simulink model "Ver1"  (R2025a)
settings: Solver=VariableStepAuto  StartTime=0.0  StopTime=50  RelTol=1e-3
model workspace (MAT data in the model file):
  params : Simulink.Parameter (value not decoded)
values from neighbouring files (symbols this model uses):
  edges = getappdata(0, 'DataEdges')    [DataAnalysis.m]    (also in Data_Analysis.m = graph_params.edges; Trajectory.m = getappdata(0, 'Edges'); data.m = graph_params.edges; formation_data.mat = [1 1 1 1 1 1 1 1 1 1 2 3 ... (62 elements, 31x2)])
  p10_init = [9; 5; 0]    [data.m]
  p2_init = [10; 0; 0]    [data.m]
  p3_init = [0; 10; 0]    [data.m]
  p4_init = [-10; 0; 0]    [data.m]
  p5_init = [0; -10; 0]    [data.m]
  p6_init = [7; 7; 0]    [data.m]
  p7_init = [-7; 7; 0]    [data.m]
  p8_init = [-7; -7; 0]    [data.m]
  p9_init = [7; -7; 0]    [data.m]
(part 2 of 3)

== matlab function Ver1/Drone 6/MATLAB Function1 ==
  data: p input; pes input; v input; u output; params parameter Bus: params_bus
function u = fcn(p, pes, v, params)

    graph_params = params.graph_params;
    formation_params = params.formation_params;
    conn_params = params.conn_params;
    avoid_params = params.avoid_params;
    prior_params = params.prior_params;

    % Chuyển vector p thành mảng 3x5
    pos = reshape(p, 3, graph_params.n_drones);
    vel = reshape(v, 3, graph_params.n_drones);
    pes = reshape(pes, 3, graph_params.n_drones);
    
    n_edges = size(graph_params.edges, 1);
    

    i_drone = 6;
    
    % =====================================================================
    %  FORMATION CONTROL (Distance-based + Backstepping)
    % =====================================================================
    u_form = zeros(3,1);
    gradV = zeros(3,1);
    dgradV = zeros(3,1);
    
    for e = 1:n_edges
        if graph_params.edges(e,1) == i_drone
            j = graph_params.edges(e,2);
            p_ij = pos(:,j) - pos(:,i_drone);
            v_ij = vel(:,j) - vel(:,i_drone);
            dij = norm(p_ij);
            
            if dij > 1e-6
                e_ij = dij^2 - formation_params.d_star(e)^2;
                
                % Lực formation (gradient descent)
                u_form = u_form + formation_params.alpha * e_ij * p_ij;
                
                % Gradient V
                gradV = gradV + e_ij * p_ij;
                
                % Đạo hàm gradient V
                term = 2*(p_ij' * v_ij) * p_ij + e_ij * v_ij;
                dgradV = dgradV + term;
            end
            
        elseif graph_params.edges(e,2) == i_drone
            j = graph_params.edges(e,1);
            p_ij = pos(:,j) - pos(:,i_drone);
            v_ij = vel(:,j) - vel(:,i_drone);
            dij = norm(p_ij);
            
            if dij > 1e-6
                e_ij = dij^2 - formation_params.d_star(e)^2;
                
                u_form = u_form + formation_params.alpha * e_ij * p_ij;
                gradV = gradV + e_ij * p_ij;
                term = 2*(p_ij' * v_ij) * p_ij + e_ij * v_ij;
                dgradV = dgradV + term;
            end
        end
    end
    
    % Giới hạn gradient
    gradV = max(min(gradV, 15), -15);
    dgradV = max(min(dgradV, 20), -20);
    
    % Backstepping
    u_back = -formation_params.kp * gradV - formation_params.kd * dgradV;
    
    % Damping
    v_i = vel(:,i_drone);
    u_damp = -formation_params.beta * v_i;
    
    % =====================================================================
    %  CONNECTIVITY MAINTENANCE
    % =====================================================================
    % Tính ma trận kề sigmoid
    A = zeros(graph_params.n_drones);
    for i = 1:graph_params.n_drones
        for j = i+1:graph_params.n_drones
            d_ij = norm(pos(:,i) - pos(:,j));
            a_ij = 1 / (1 + exp(-conn_params.omega * (conn_params.d_max - d_ij)));
            A(i,j) = a_ij;
            A(j,i) = a_ij;
        end
    end
    
    % Ma trận Laplace
    D = diag(sum(A,2));
    L = D - A;
    
    % Tính M = Q'*L*Q
    Q = conn_params.Q;
    M = Q' * L * Q;
    lambda2 = min(eig(M));
    
    detM = det(M);
    if detM < 1e-6
        detM = 1e-6;
    end
    
    % Tính lực giữ liên kết bằng sai phân số
    u_conn = zeros(3, 1);
    eps_fd = 1e-4;
    
    for d = 1:graph_params.dim
        % M tại p + eps
        pos_plus = pos;
        pos_plus(d, i_drone) = pos_plus(d, i_drone) + eps_fd;
        
        A_plus = zeros(graph_params.n_drones);
        for i = 1:graph_params.n_drones
            for j = i+1:graph_params.n_drones
                d_ij = norm(pos_plus(:,i) - pos_plus(:,j));
                a_ij = 1 / (1 + exp(-conn_params.omega * (conn_params.d_max - d_ij)));
                A_plus(i,j) = a_ij;
                A_plus(j,i) = a_ij;
            end
        end
        D_plus = diag(sum(A_plus,2));
        L_plus = D_plus - A_plus;
        M_plus = Q' * L_plus * Q;
        
        % M tại p - eps
        pos_minus = pos;
        pos_minus(d, i_drone) = pos_minus(d, i_drone) - eps_fd;
        
        A_minus = zeros(graph_params.n_drones);
        for i = 1:graph_params.n_drones
            for j = i+1:graph_params.n_drones
                d_ij = norm(pos_minus(:,i) - pos_minus(:,j));
                a_ij = 1 / (1 + exp(-conn_params.omega * (conn_params.d_max - d_ij)));
                A_minus(i,j) = a_ij;
                A_minus(j,i) = a_ij;
            end
        end
        D_minus = diag(sum(A_minus,2));
        L_minus = D_minus - A_minus;
        M_minus = Q' * L_minus * Q;
        
        dM_dp = (M_plus - M_minus) / (2*eps_fd);
        
        if rcond(M) > 1e-6
            u_conn(d) = conn_params.alpha * trace(M \ dM_dp) / detM^conn_params.alpha;
        else
            u_conn(d) = 0;
        end
    end
    
    % =====================================================================
    %  OBSTACLE AVOIDANCE
    % =====================================================================
    muy = (1 + avoid_params.d_safe^4) / avoid_params.d_safe^4;
    
    % Tính beta_product
    beta_product = 1;
    for e = 1:n_edges
        i = graph_params.edges(e,1);
        j = graph_params.edges(e,2);
        dij = norm(pos(:,i) - pos(:,j));
        beta_val = beta_slide(dij, avoid_params.d_safe, muy);
        beta_product = beta_product * beta_val;
    end
    
    Phi = 1 / (beta_product^avoid_params.alpha);
    dPhi_dbeta = -avoid_params.alpha * beta_product^(-avoid_params.alpha-1);
    
    % Tính lực tránh
    u_avoid = zeros(3, 1);
    eps_deriv = 1e-4;
    
    for j = 1:graph_params.n_drones
        if j == i_drone
            continue;
        end
        
        p_ij = pos(:,i_drone) - pos(:,j);
        dij_ij = norm(p_ij);
        
        if dij_ij > 1e-6
            dd_dp = p_ij;
            
            % Đạo hàm số của beta
            beta_plus = beta_slide(dij_ij + eps_deriv, avoid_params.d_safe, muy);
            beta_minus = beta_slide(dij_ij - eps_deriv, avoid_params.d_safe, muy);
            dbeta_dd = (beta_plus - beta_minus) / (2*eps_deriv);
            
            grad = dPhi_dbeta * dbeta_dd * dd_dp;
            u_avoid = u_avoid - avoid_params.k * grad;
        end
    end
    
    u_h = [0; 0; -prior_params.k_height * (pes(3, i_drone) - pos(3, 1))];


    % =====================================================================
    %  TỔNG HỢP
    % =====================================================================
    u = 5*u_form + u_back + u_damp + 0.5*u_conn + 10*u_avoid + u_h;

end

function beta = beta_slide(dist, d_safe, muy)
    if (dist^2 - d_safe^2) >= 0
        rho = 0;
    else
        rho = 1;
    end
    diff_sq = (dist^2 - d_safe^2)^2;
    beta = (1 - muy * diff_sq / (1 + diff_sq))^rho;
    % Đảm bảo beta không âm
    beta = max(beta, 0);
end

== matlab function Ver1/Drone 6/Pos Estimation ==
  data: p input; v input; pes input; pes_dot output size=[3,1]; params parameter Bus: params_bus
function pes_dot = fcn(p, v, pes, params)

    graph_params = params.graph_params;
    estimation_params = params.estimation_params;

    pes_dot = zeros(3,1);
    
    
    i_drone = 6;  % Drone đang xét
    
    % Reshape input
    pos = reshape(p, graph_params.dim, graph_params.n_drones);
    pes = reshape(pes, graph_params.dim, graph_params.n_drones);
    vel = reshape(v, graph_params.dim, graph_params.n_drones);
    
    % Tính toán gradient term
    grad_term = zeros(graph_params.dim, 1);
    
    n_edges = size(graph_params.edges, 1);
    
    for e = 1:n_edges
        if graph_params.edges(e,1) == i_drone
            j = graph_params.edges(e,2);
        else
            j = graph_params.edges(e,1);
        end

        if j == 1
            grad_term = grad_term + ((pos(:, j) - pes(:,i_drone)) - (pos(:, j) - pos(:, i_drone)));
        else
            grad_term = grad_term + (pes(:, j) - pes(:, i_drone) - (pos(:, j) - pos(:, i_drone)));
        end
    end

    
    % Output
    
    pes_dot1 = vel(:, i_drone) + estimation_params.mu*grad_term;
    pes_dot = [pes_dot1(1); pes_dot1(2); pes_dot1(3)];
end

== matlab function Ver1/Drone 6/Subsystem/Kinematic ==
  data: p_ddot output; u input
function p_ddot = fcn(u)

    p_ddot = u;

end

== matlab function Ver1/Drone 7/MATLAB Function1 ==
  data: p input; pes input; v input; u output; params parameter Bus: params_bus
function u = fcn(p, pes, v, params)

    graph_params = params.graph_params;
    formation_params = params.formation_params;
    conn_params = params.conn_params;
    avoid_params = params.avoid_params;
    prior_params = params.prior_params;

    % Chuyển vector p thành mảng 3x5
    pos = reshape(p, 3, graph_params.n_drones);
    vel = reshape(v, 3, graph_params.n_drones);
    pes = reshape(pes, 3, graph_params.n_drones);
    
    n_edges = size(graph_params.edges, 1);
    

    i_drone = 7;
    
    % =====================================================================
    %  FORMATION CONTROL (Distance-based + Backstepping)
    % =====================================================================
    u_form = zeros(3,1);
    gradV = zeros(3,1);
    dgradV = zeros(3,1);
    
    for e = 1:n_edges
        if graph_params.edges(e,1) == i_drone
            j = graph_params.edges(e,2);
            p_ij = pos(:,j) - pos(:,i_drone);
            v_ij = vel(:,j) - vel(:,i_drone);
            dij = norm(p_ij);
            
            if dij > 1e-6
                e_ij = dij^2 - formation_params.d_star(e)^2;
                
                % Lực formation (gradient descent)
                u_form = u_form + formation_params.alpha * e_ij * p_ij;
                
                % Gradient V
                gradV = gradV + e_ij * p_ij;
                
                % Đạo hàm gradient V
                term = 2*(p_ij' * v_ij) * p_ij + e_ij * v_ij;
                dgradV = dgradV + term;
            end
            
        elseif graph_params.edges(e,2) == i_drone
            j = graph_params.edges(e,1);
            p_ij = pos(:,j) - pos(:,i_drone);
            v_ij = vel(:,j) - vel(:,i_drone);
            dij = norm(p_ij);
            
            if dij > 1e-6
                e_ij = dij^2 - formation_params.d_star(e)^2;
                
                u_form = u_form + formation_params.alpha * e_ij * p_ij;
                gradV = gradV + e_ij * p_ij;
                term = 2*(p_ij' * v_ij) * p_ij + e_ij * v_ij;
                dgradV = dgradV + term;
            end
        end
    end
    
    % Giới hạn gradient
    gradV = max(min(gradV, 15), -15);
    dgradV = max(min(dgradV, 20), -20);
    
    % Backstepping
    u_back = -formation_params.kp * gradV - formation_params.kd * dgradV;
    
    % Damping
    v_i = vel(:,i_drone);
    u_damp = -formation_params.beta * v_i;
    
    % =====================================================================
    %  CONNECTIVITY MAINTENANCE
    % =====================================================================
    % Tính ma trận kề sigmoid
    A = zeros(graph_params.n_drones);
    for i = 1:graph_params.n_drones
        for j = i+1:graph_params.n_drones
            d_ij = norm(pos(:,i) - pos(:,j));
            a_ij = 1 / (1 + exp(-conn_params.omega * (conn_params.d_max - d_ij)));
            A(i,j) = a_ij;
            A(j,i) = a_ij;
        end
    end
    
    % Ma trận Laplace
    D = diag(sum(A,2));
    L = D - A;
    
    % Tính M = Q'*L*Q
    Q = conn_params.Q;
    M = Q' * L * Q;
    lambda2 = min(eig(M));
    
    detM = det(M);
    if detM < 1e-6
        detM = 1e-6;
    end
    
    % Tính lực giữ liên kết bằng sai phân số
    u_conn = zeros(3, 1);
    eps_fd = 1e-4;
    
    for d = 1:graph_params.dim
        % M tại p + eps
        pos_plus = pos;
        pos_plus(d, i_drone) = pos_plus(d, i_drone) + eps_fd;
        
        A_plus = zeros(graph_params.n_drones);
        for i = 1:graph_params.n_drones
            for j = i+1:graph_params.n_drones
                d_ij = norm(pos_plus(:,i) - pos_plus(:,j));
                a_ij = 1 / (1 + exp(-conn_params.omega * (conn_params.d_max - d_ij)));
                A_plus(i,j) = a_ij;
                A_plus(j,i) = a_ij;
            end
        end
        D_plus = diag(sum(A_plus,2));
        L_plus = D_plus - A_plus;
        M_plus = Q' * L_plus * Q;
        
        % M tại p - eps
        pos_minus = pos;
        pos_minus(d, i_drone) = pos_minus(d, i_drone) - eps_fd;
        
        A_minus = zeros(graph_params.n_drones);
        for i = 1:graph_params.n_drones
            for j = i+1:graph_params.n_drones
                d_ij = norm(pos_minus(:,i) - pos_minus(:,j));
                a_ij = 1 / (1 + exp(-conn_params.omega * (conn_params.d_max - d_ij)));
                A_minus(i,j) = a_ij;
                A_minus(j,i) = a_ij;
            end
        end
        D_minus = diag(sum(A_minus,2));
        L_minus = D_minus - A_minus;
        M_minus = Q' * L_minus * Q;
        
        dM_dp = (M_plus - M_minus) / (2*eps_fd);
        
        if rcond(M) > 1e-6
            u_conn(d) = conn_params.alpha * trace(M \ dM_dp) / detM^conn_params.alpha;
        else
            u_conn(d) = 0;
        end
    end
    
    % =====================================================================
    %  OBSTACLE AVOIDANCE
    % =====================================================================
    muy = (1 + avoid_params.d_safe^4) / avoid_params.d_safe^4;
    
    % Tính beta_product
    beta_product = 1;
    for e = 1:n_edges
        i = graph_params.edges(e,1);
        j = graph_params.edges(e,2);
        dij = norm(pos(:,i) - pos(:,j));
        beta_val = beta_slide(dij, avoid_params.d_safe, muy);
        beta_product = beta_product * beta_val;
    end
    
    Phi = 1 / (beta_product^avoid_params.alpha);
    dPhi_dbeta = -avoid_params.alpha * beta_product^(-avoid_params.alpha-1);
    
    % Tính lực tránh
    u_avoid = zeros(3, 1);
    eps_deriv = 1e-4;
    
    for j = 1:graph_params.n_drones
        if j == i_drone
            continue;
        end
        
        p_ij = pos(:,i_drone) - pos(:,j);
        dij_ij = norm(p_ij);
        
        if dij_ij > 1e-6
            dd_dp = p_ij;
            
            % Đạo hàm số của beta
            beta_plus = beta_slide(dij_ij + eps_deriv, avoid_params.d_safe, muy);
            beta_minus = beta_slide(dij_ij - eps_deriv, avoid_params.d_safe, muy);
            dbeta_dd = (beta_plus - beta_minus) / (2*eps_deriv);
            
            grad = dPhi_dbeta * dbeta_dd * dd_dp;
            u_avoid = u_avoid - avoid_params.k * grad;
        end
    end
    
    u_h = [0; 0; -prior_params.k_height * (pes(3, i_drone) - pos(3, 1))];


    % =====================================================================
    %  TỔNG HỢP
    % =====================================================================
    u = 5*u_form + u_back + u_damp + 0.5*u_conn + 10*u_avoid + u_h;

end

function beta = beta_slide(dist, d_safe, muy)
    if (dist^2 - d_safe^2) >= 0
        rho = 0;
    else
        rho = 1;
    end
    diff_sq = (dist^2 - d_safe^2)^2;
    beta = (1 - muy * diff_sq / (1 + diff_sq))^rho;
    % Đảm bảo beta không âm
    beta = max(beta, 0);
end

== matlab function Ver1/Drone 7/Pos Estimation ==
  data: p input; v input; pes input; pes_dot output size=[3,1]; params parameter Bus: params_bus
function pes_dot = fcn(p, v, pes, params)

    graph_params = params.graph_params;
    estimation_params = params.estimation_params;

    pes_dot = zeros(3,1);
    
    
    i_drone = 7;  % Drone đang xét
    
    % Reshape input
    pos = reshape(p, graph_params.dim, graph_params.n_drones);
    pes = reshape(pes, graph_params.dim, graph_params.n_drones);
    vel = reshape(v, graph_params.dim, graph_params.n_drones);
    
    % Tính toán gradient term
    grad_term = zeros(graph_params.dim, 1);
    
    n_edges = size(graph_params.edges, 1);
    
    for e = 1:n_edges
        if graph_params.edges(e,1) == i_drone
            j = graph_params.edges(e,2);
        else
            j = graph_params.edges(e,1);
        end

        if j == 1
            grad_term = grad_term + ((pos(:, j) - pes(:,i_drone)) - (pos(:, j) - pos(:, i_drone)));
        else
            grad_term = grad_term + (pes(:, j) - pes(:, i_drone) - (pos(:, j) - pos(:, i_drone)));
        end
    end

    
    % Output
    
    pes_dot1 = vel(:, i_drone) + estimation_params.mu*grad_term;
    pes_dot = [pes_dot1(1); pes_dot1(2); pes_dot1(3)];
end

== matlab function Ver1/Drone 7/Subsystem/Kinematic ==
  data: p_ddot output; u input
function p_ddot = fcn(u)

    p_ddot = u;

end

== matlab function Ver1/Drone 8/MATLAB Function1 ==
  data: p input; pes input; v input; u output; params parameter Bus: params_bus
function u = fcn(p, pes, v, params)

    graph_params = params.graph_params;
    formation_params = params.formation_params;
    conn_params = params.conn_params;
    avoid_params = params.avoid_params;
    prior_params = params.prior_params;

    % Chuyển vector p thành mảng 3x5
    pos = reshape(p, 3, graph_params.n_drones);
    vel = reshape(v, 3, graph_params.n_drones);
    pes = reshape(pes, 3, graph_params.n_drones);
    
    n_edges = size(graph_params.edges, 1);
    

    i_drone = 8;
    
    % =====================================================================
    %  FORMATION CONTROL (Distance-based + Backstepping)
    % =====================================================================
    u_form = zeros(3,1);
    gradV = zeros(3,1);
    dgradV = zeros(3,1);
    
    for e = 1:n_edges
        if graph_params.edges(e,1) == i_drone
            j = graph_params.edges(e,2);
            p_ij = pos(:,j) - pos(:,i_drone);
            v_ij = vel(:,j) - vel(:,i_drone);
            dij = norm(p_ij);
            
            if dij > 1e-6
                e_ij = dij^2 - formation_params.d_star(e)^2;
                
                % Lực formation (gradient descent)
                u_form = u_form + formation_params.alpha * e_ij * p_ij;
                
                % Gradient V
                gradV = gradV + e_ij * p_ij;
                
                % Đạo hàm gradient V
                term = 2*(p_ij' * v_ij) * p_ij + e_ij * v_ij;
                dgradV = dgradV + term;
            end
            
        elseif graph_params.edges(e,2) == i_drone
            j = graph_params.edges(e,1);
            p_ij = pos(:,j) - pos(:,i_drone);
            v_ij = vel(:,j) - vel(:,i_drone);
            dij = norm(p_ij);
            
            if dij > 1e-6
                e_ij = dij^2 - formation_params.d_star(e)^2;
                
                u_form = u_form + formation_params.alpha * e_ij * p_ij;
                gradV = gradV + e_ij * p_ij;
                term = 2*(p_ij' * v_ij) * p_ij + e_ij * v_ij;
                dgradV = dgradV + term;
            end
        end
    end
    
    % Giới hạn gradient
    gradV = max(min(gradV, 15), -15);
    dgradV = max(min(dgradV, 20), -20);
    
    % Backstepping
    u_back = -formation_params.kp * gradV - formation_params.kd * dgradV;
    
    % Damping
    v_i = vel(:,i_drone);
    u_damp = -formation_params.beta * v_i;
    
    % =====================================================================
    %  CONNECTIVITY MAINTENANCE
    % =====================================================================
    % Tính ma trận kề sigmoid
    A = zeros(graph_params.n_drones);
    for i = 1:graph_params.n_drones
        for j = i+1:graph_params.n_drones
            d_ij = norm(pos(:,i) - pos(:,j));
            a_ij = 1 / (1 + exp(-conn_params.omega * (conn_params.d_max - d_ij)));
            A(i,j) = a_ij;
            A(j,i) = a_ij;
        end
    end
    
    % Ma trận Laplace
    D = diag(sum(A,2));
    L = D - A;
    
    % Tính M = Q'*L*Q
    Q = conn_params.Q;
    M = Q' * L * Q;
    lambda2 = min(eig(M));
    
    detM = det(M);
    if detM < 1e-6
        detM = 1e-6;
    end
    
    % Tính lực giữ liên kết bằng sai phân số
    u_conn = zeros(3, 1);
    eps_fd = 1e-4;
    
    for d = 1:graph_params.dim
        % M tại p + eps
        pos_plus = pos;
        pos_plus(d, i_drone) = pos_plus(d, i_drone) + eps_fd;
        
        A_plus = zeros(graph_params.n_drones);
        for i = 1:graph_params.n_drones
            for j = i+1:graph_params.n_drones
                d_ij = norm(pos_plus(:,i) - pos_plus(:,j));
                a_ij = 1 / (1 + exp(-conn_params.omega * (conn_params.d_max - d_ij)));
                A_plus(i,j) = a_ij;
                A_plus(j,i) = a_ij;
            end
        end
        D_plus = diag(sum(A_plus,2));
        L_plus = D_plus - A_plus;
        M_plus = Q' * L_plus * Q;
        
        % M tại p - eps
        pos_minus = pos;
        pos_minus(d, i_drone) = pos_minus(d, i_drone) - eps_fd;
        
        A_minus = zeros(graph_params.n_drones);
        for i = 1:graph_params.n_drones
            for j = i+1:graph_params.n_drones
                d_ij = norm(pos_minus(:,i) - pos_minus(:,j));
                a_ij = 1 / (1 + exp(-conn_params.omega * (conn_params.d_max - d_ij)));
                A_minus(i,j) = a_ij;
                A_minus(j,i) = a_ij;
            end
        end
        D_minus = diag(sum(A_minus,2));
        L_minus = D_minus - A_minus;
        M_minus = Q' * L_minus * Q;
        
        dM_dp = (M_plus - M_minus) / (2*eps_fd);
        
        if rcond(M) > 1e-6
            u_conn(d) = conn_params.alpha * trace(M \ dM_dp) / detM^conn_params.alpha;
        else
            u_conn(d) = 0;
        end
    end
    
    % =====================================================================
    %  OBSTACLE AVOIDANCE
    % =====================================================================
    muy = (1 + avoid_params.d_safe^4) / avoid_params.d_safe^4;
    
    % Tính beta_product
    beta_product = 1;
    for e = 1:n_edges
        i = graph_params.edges(e,1);
        j = graph_params.edges(e,2);
        dij = norm(pos(:,i) - pos(:,j));
        beta_val = beta_slide(dij, avoid_params.d_safe, muy);
        beta_product = beta_product * beta_val;
    end
    
    Phi = 1 / (beta_product^avoid_params.alpha);
    dPhi_dbeta = -avoid_params.alpha * beta_product^(-avoid_params.alpha-1);
    
    % Tính lực tránh
    u_avoid = zeros(3, 1);
    eps_deriv = 1e-4;
    
    for j = 1:graph_params.n_drones
        if j == i_drone
            continue;
        end
        
        p_ij = pos(:,i_drone) - pos(:,j);
        dij_ij = norm(p_ij);
        
        if dij_ij > 1e-6
            dd_dp = p_ij;
            
            % Đạo hàm số của beta
            beta_plus = beta_slide(dij_ij + eps_deriv, avoid_params.d_safe, muy);
            beta_minus = beta_slide(dij_ij - eps_deriv, avoid_params.d_safe, muy);
            dbeta_dd = (beta_plus - beta_minus) / (2*eps_deriv);
            
            grad = dPhi_dbeta * dbeta_dd * dd_dp;
            u_avoid = u_avoid - avoid_params.k * grad;
        end
    end
    
    u_h = [0; 0; -prior_params.k_height * (pes(3, i_drone) - pos(3, 1))];


    % =====================================================================
    %  TỔNG HỢP
    % =====================================================================
    u = 5*u_form + u_back + u_damp + 0.5*u_conn + 10*u_avoid + u_h;

end

function beta = beta_slide(dist, d_safe, muy)
    if (dist^2 - d_safe^2) >= 0
        rho = 0;
    else
        rho = 1;
    end
    diff_sq = (dist^2 - d_safe^2)^2;
    beta = (1 - muy * diff_sq / (1 + diff_sq))^rho;
    % Đảm bảo beta không âm
    beta = max(beta, 0);
end

== matlab function Ver1/Drone 8/Pos Estimation ==
  data: p input; v input; pes input; pes_dot output size=[3,1]; params parameter Bus: params_bus
function pes_dot = fcn(p, v, pes, params)

    graph_params = params.graph_params;
    estimation_params = params.estimation_params;

    pes_dot = zeros(3,1);
    
    
    i_drone = 8;  % Drone đang xét
    
    % Reshape input
    pos = reshape(p, graph_params.dim, graph_params.n_drones);
    pes = reshape(pes, graph_params.dim, graph_params.n_drones);
    vel = reshape(v, graph_params.dim, graph_params.n_drones);
    
    % Tính toán gradient term
    grad_term = zeros(graph_params.dim, 1);
    
    n_edges = size(graph_params.edges, 1);
    
    for e = 1:n_edges
        if graph_params.edges(e,1) == i_drone
            j = graph_params.edges(e,2);
        else
            j = graph_params.edges(e,1);
        end

        if j == 1
            grad_term = grad_term + ((pos(:, j) - pes(:,i_drone)) - (pos(:, j) - pos(:, i_drone)));
        else
            grad_term = grad_term + (pes(:, j) - pes(:, i_drone) - (pos(:, j) - pos(:, i_drone)));
        end
    end

    
    % Output
    
    pes_dot1 = vel(:, i_drone) + estimation_params.mu*grad_term;
    pes_dot = [pes_dot1(1); pes_dot1(2); pes_dot1(3)];
end

== matlab function Ver1/Drone 8/Subsystem/Kinematic ==
  data: p_ddot output; u input
function p_ddot = fcn(u)

    p_ddot = u;

end

== matlab function Ver1/Drone 9/MATLAB Function1 ==
  data: p input; pes input; v input; u output; params parameter Bus: params_bus
function u = fcn(p, pes, v, params)

    graph_params = params.graph_params;
    formation_params = params.formation_params;
    conn_params = params.conn_params;
    avoid_params = params.avoid_params;
    prior_params = params.prior_params;

    % Chuyển vector p thành mảng 3x5
    pos = reshape(p, 3, graph_params.n_drones);
    vel = reshape(v, 3, graph_params.n_drones);
    pes = reshape(pes, 3, graph_params.n_drones);
    
    n_edges = size(graph_params.edges, 1);
    

    i_drone = 9;
    
    % =====================================================================
    %  FORMATION CONTROL (Distance-based + Backstepping)
    % =====================================================================
    u_form = zeros(3,1);
    gradV = zeros(3,1);
    dgradV = zeros(3,1);
    
    for e = 1:n_edges
        if graph_params.edges(e,1) == i_drone
            j = graph_params.edges(e,2);
            p_ij = pos(:,j) - pos(:,i_drone);
            v_ij = vel(:,j) - vel(:,i_drone);
            dij = norm(p_ij);
            
            if dij > 1e-6
                e_ij = dij^2 - formation_params.d_star(e)^2;
                
                % Lực formation (gradient descent)
                u_form = u_form + formation_params.alpha * e_ij * p_ij;
                
                % Gradient V
                gradV = gradV + e_ij * p_ij;
                
                % Đạo hàm gradient V
                term = 2*(p_ij' * v_ij) * p_ij + e_ij * v_ij;
                dgradV = dgradV + term;
            end
            
        elseif graph_params.edges(e,2) == i_drone
            j = graph_params.edges(e,1);
            p_ij = pos(:,j) - pos(:,i_drone);
            v_ij = vel(:,j) - vel(:,i_drone);
            dij = norm(p_ij);
            
            if dij > 1e-6
                e_ij = dij^2 - formation_params.d_star(e)^2;
                
                u_form = u_form + formation_params.alpha * e_ij * p_ij;
                gradV = gradV + e_ij * p_ij;
                term = 2*(p_ij' * v_ij) * p_ij + e_ij * v_ij;
                dgradV = dgradV + term;
            end
        end
    end
    
    % Giới hạn gradient
    gradV = max(min(gradV, 15), -15);
    dgradV = max(min(dgradV, 20), -20);
    
    % Backstepping
    u_back = -formation_params.kp * gradV - formation_params.kd * dgradV;
    
    % Damping
    v_i = vel(:,i_drone);
    u_damp = -formation_params.beta * v_i;
    
    % =====================================================================
    %  CONNECTIVITY MAINTENANCE
    % =====================================================================
    % Tính ma trận kề sigmoid
    A = zeros(graph_params.n_drones);
    for i = 1:graph_params.n_drones
        for j = i+1:graph_params.n_drones
            d_ij = norm(pos(:,i) - pos(:,j));
            a_ij = 1 / (1 + exp(-conn_params.omega * (conn_params.d_max - d_ij)));
            A(i,j) = a_ij;
            A(j,i) = a_ij;
        end
    end
    
    % Ma trận Laplace
    D = diag(sum(A,2));
    L = D - A;
    
    % Tính M = Q'*L*Q
    Q = conn_params.Q;
    M = Q' * L * Q;
    lambda2 = min(eig(M));
    
    detM = det(M);
    if detM < 1e-6
        detM = 1e-6;
    end
    
    % Tính lực giữ liên kết bằng sai phân số
    u_conn = zeros(3, 1);
    eps_fd = 1e-4;
    
    for d = 1:graph_params.dim
        % M tại p + eps
        pos_plus = pos;
        pos_plus(d, i_drone) = pos_plus(d, i_drone) + eps_fd;
        
        A_plus = zeros(graph_params.n_drones);
        for i = 1:graph_params.n_drones
            for j = i+1:graph_params.n_drones
                d_ij = norm(pos_plus(:,i) - pos_plus(:,j));
                a_ij = 1 / (1 + exp(-conn_params.omega * (conn_params.d_max - d_ij)));
                A_plus(i,j) = a_ij;
                A_plus(j,i) = a_ij;
            end
        end
        D_plus = diag(sum(A_plus,2));
        L_plus = D_plus - A_plus;
        M_plus = Q' * L_plus * Q;
        
        % M tại p - eps
        pos_minus = pos;
        pos_minus(d, i_drone) = pos_minus(d, i_drone) - eps_fd;
        
        A_minus = zeros(graph_params.n_drones);
        for i = 1:graph_params.n_drones
            for j = i+1:graph_params.n_drones
                d_ij = norm(pos_minus(:,i) - pos_minus(:,j));
                a_ij = 1 / (1 + exp(-conn_params.omega * (conn_params.d_max - d_ij)));
                A_minus(i,j) = a_ij;
                A_minus(j,i) = a_ij;
            end
        end
        D_minus = diag(sum(A_minus,2));
        L_minus = D_minus - A_minus;
        M_minus = Q' * L_minus * Q;
        
        dM_dp = (M_plus - M_minus) / (2*eps_fd);
        
        if rcond(M) > 1e-6
            u_conn(d) = conn_params.alpha * trace(M \ dM_dp) / detM^conn_params.alpha;
        else
            u_conn(d) = 0;
        end
    end
    
    % =====================================================================
    %  OBSTACLE AVOIDANCE
    % =====================================================================
    muy = (1 + avoid_params.d_safe^4) / avoid_params.d_safe^4;
    
    % Tính beta_product
    beta_product = 1;
    for e = 1:n_edges
        i = graph_params.edges(e,1);
        j = graph_params.edges(e,2);
        dij = norm(pos(:,i) - pos(:,j));
        beta_val = beta_slide(dij, avoid_params.d_safe, muy);
        beta_product = beta_product * beta_val;
    end
    
    Phi = 1 / (beta_product^avoid_params.alpha);
    dPhi_dbeta = -avoid_params.alpha * beta_product^(-avoid_params.alpha-1);
    
    % Tính lực tránh
    u_avoid = zeros(3, 1);
    eps_deriv = 1e-4;
    
    for j = 1:graph_params.n_drones
        if j == i_drone
            continue;
        end
        
        p_ij = pos(:,i_drone) - pos(:,j);
        dij_ij = norm(p_ij);
        
        if dij_ij > 1e-6
            dd_dp = p_ij;
            
            % Đạo hàm số của beta
            beta_plus = beta_slide(dij_ij + eps_deriv, avoid_params.d_safe, muy);
            beta_minus = beta_slide(dij_ij - eps_deriv, avoid_params.d_safe, muy);
            dbeta_dd = (beta_plus - beta_minus) / (2*eps_deriv);
            
            grad = dPhi_dbeta * dbeta_dd * dd_dp;
            u_avoid = u_avoid - avoid_params.k * grad;
        end
    end
    
    u_h = [0; 0; -prior_params.k_height * (pes(3, i_drone) - pos(3, 1))];


    % =====================================================================
    %  TỔNG HỢP
    % =====================================================================
    u = 5*u_form + u_back + u_damp + 0.5*u_conn + 10*u_avoid + u_h;

end

function beta = beta_slide(dist, d_safe, muy)
    if (dist^2 - d_safe^2) >= 0
        rho = 0;
    else
        rho = 1;
    end
    diff_sq = (dist^2 - d_safe^2)^2;
    beta = (1 - muy * diff_sq / (1 + diff_sq))^rho;
    % Đảm bảo beta không âm
    beta = max(beta, 0);
end

== matlab function Ver1/Drone 9/Pos Estimation ==
  data: p input; v input; pes input; pes_dot output size=[3,1]; params parameter Bus: params_bus
function pes_dot = fcn(p, v, pes, params)

    graph_params = params.graph_params;
    estimation_params = params.estimation_params;

    pes_dot = zeros(3,1);
    
    
    i_drone = 9;  % Drone đang xét
    
    % Reshape input
    pos = reshape(p, graph_params.dim, graph_params.n_drones);
    pes = reshape(pes, graph_params.dim, graph_params.n_drones);
    vel = reshape(v, graph_params.dim, graph_params.n_drones);
    
    % Tính toán gradient term
    grad_term = zeros(graph_params.dim, 1);
    
    n_edges = size(graph_params.edges, 1);
    
    for e = 1:n_edges
        if graph_params.edges(e,1) == i_drone
            j = graph_params.edges(e,2);
        else
            j = graph_params.edges(e,1);
        end

        if j == 1
            grad_term = grad_term + ((pos(:, j) - pes(:,i_drone)) - (pos(:, j) - pos(:, i_drone)));
        else
            grad_term = grad_term + (pes(:, j) - pes(:, i_drone) - (pos(:, j) - pos(:, i_drone)));
        end
    end

    
    % Output
    
    pes_dot1 = vel(:, i_drone) + estimation_params.mu*grad_term;
    pes_dot = [pes_dot1(1); pes_dot1(2); pes_dot1(3)];
end

== matlab function Ver1/Drone 9/Subsystem/Kinematic ==
  data: p_ddot output; u input
function p_ddot = fcn(u)

    p_ddot = u;

end

== matlab function Ver1/Drone 10/MATLAB Function1 ==
  data: p input; pes input; v input; u output; params parameter Bus: params_bus
function u = fcn(p, pes, v, params)

    graph_params = params.graph_params;
    formation_params = params.formation_params;
    conn_params = params.conn_params;
    avoid_params = params.avoid_params;
    prior_params = params.prior_params;

    % Chuyển vector p thành mảng 3x5
    pos = reshape(p, 3, graph_params.n_drones);
    vel = reshape(v, 3, graph_params.n_drones);
    pes = reshape(pes, 3, graph_params.n_drones);
    
    n_edges = size(graph_params.edges, 1);
    

    i_drone = 10;
    
    % =====================================================================
    %  FORMATION CONTROL (Distance-based + Backstepping)
    % =====================================================================
    u_form = zeros(3,1);
    gradV = zeros(3,1);
    dgradV = zeros(3,1);
    
    for e = 1:n_edges
        if graph_params.edges(e,1) == i_drone
            j = graph_params.edges(e,2);
            p_ij = pos(:,j) - pos(:,i_drone);
            v_ij = vel(:,j) - vel(:,i_drone);
            dij = norm(p_ij);
            
            if dij > 1e-6
                e_ij = dij^2 - formation_params.d_star(e)^2;
                
                % Lực formation (gradient descent)
                u_form = u_form + formation_params.alpha * e_ij * p_ij;
                
                % Gradient V
                gradV = gradV + e_ij * p_ij;
                
                % Đạo hàm gradient V
                term = 2*(p_ij' * v_ij) * p_ij + e_ij * v_ij;
                dgradV = dgradV + term;
            end
            
        elseif graph_params.edges(e,2) == i_drone
            j = graph_params.edges(e,1);
            p_ij = pos(:,j) - pos(:,i_drone);
            v_ij = vel(:,j) - vel(:,i_drone);
            dij = norm(p_ij);
            
            if dij > 1e-6
                e_ij = dij^2 - formation_params.d_star(e)^2;
                
                u_form = u_form + formation_params.alpha * e_ij * p_ij;
                gradV = gradV + e_ij * p_ij;
                term = 2*(p_ij' * v_ij) * p_ij + e_ij * v_ij;
                dgradV = dgradV + term;
            end
        end
    end
    
    % Giới hạn gradient
    gradV = max(min(gradV, 15), -15);
    dgradV = max(min(dgradV, 20), -20);
    
    % Backstepping
    u_back = -formation_params.kp * gradV - formation_params.kd * dgradV;
    
    % Damping
    v_i = vel(:,i_drone);
    u_damp = -formation_params.beta * v_i;
    
    % =====================================================================
    %  CONNECTIVITY MAINTENANCE
    % =====================================================================
    % Tính ma trận kề sigmoid
    A = zeros(graph_params.n_drones);
    for i = 1:graph_params.n_drones
        for j = i+1:graph_params.n_drones
            d_ij = norm(pos(:,i) - pos(:,j));
            a_ij = 1 / (1 + exp(-conn_params.omega * (conn_params.d_max - d_ij)));
            A(i,j) = a_ij;
            A(j,i) = a_ij;
        end
    end
    
    % Ma trận Laplace
    D = diag(sum(A,2));
    L = D - A;
    
    % Tính M = Q'*L*Q
    Q = conn_params.Q;
    M = Q' * L * Q;
    lambda2 = min(eig(M));
    
    detM = det(M);
    if detM < 1e-6
        detM = 1e-6;
    end
    
    % Tính lực giữ liên kết bằng sai phân số
    u_conn = zeros(3, 1);
    eps_fd = 1e-4;
    
    for d = 1:graph_params.dim
        % M tại p + eps
        pos_plus = pos;
        pos_plus(d, i_drone) = pos_plus(d, i_drone) + eps_fd;
        
        A_plus = zeros(graph_params.n_drones);
        for i = 1:graph_params.n_drones
            for j = i+1:graph_params.n_drones
                d_ij = norm(pos_plus(:,i) - pos_plus(:,j));
                a_ij = 1 / (1 + exp(-conn_params.omega * (conn_params.d_max - d_ij)));
                A_plus(i,j) = a_ij;
                A_plus(j,i) = a_ij;
            end
        end
        D_plus = diag(sum(A_plus,2));
        L_plus = D_plus - A_plus;
        M_plus = Q' * L_plus * Q;
        
        % M tại p - eps
        pos_minus = pos;
        pos_minus(d, i_drone) = pos_minus(d, i_drone) - eps_fd;
        
        A_minus = zeros(graph_params.n_drones);
        for i = 1:graph_params.n_drones
            for j = i+1:graph_params.n_drones
                d_ij = norm(pos_minus(:,i) - pos_minus(:,j));
                a_ij = 1 / (1 + exp(-conn_params.omega * (conn_params.d_max - d_ij)));
                A_minus(i,j) = a_ij;
                A_minus(j,i) = a_ij;
            end
        end
        D_minus = diag(sum(A_minus,2));
        L_minus = D_minus - A_minus;
        M_minus = Q' * L_minus * Q;
        
        dM_dp = (M_plus - M_minus) / (2*eps_fd);
        
        if rcond(M) > 1e-6
            u_conn(d) = conn_params.alpha * trace(M \ dM_dp) / detM^conn_params.alpha;
        else
            u_conn(d) = 0;
        end
    end
    
    % =====================================================================
    %  OBSTACLE AVOIDANCE
    % =====================================================================
    muy = (1 + avoid_params.d_safe^4) / avoid_params.d_safe^4;
    
    % Tính beta_product
    beta_product = 1;
    for e = 1:n_edges
        i = graph_params.edges(e,1);
        j = graph_params.edges(e,2);
        dij = norm(pos(:,i) - pos(:,j));
        beta_val = beta_slide(dij, avoid_params.d_safe, muy);
        beta_product = beta_product * beta_val;
    end
    
    Phi = 1 / (beta_product^avoid_params.alpha);
    dPhi_dbeta = -avoid_params.alpha * beta_product^(-avoid_params.alpha-1);
    
    % Tính lực tránh
    u_avoid = zeros(3, 1);
    eps_deriv = 1e-4;
    
    for j = 1:graph_params.n_drones
        if j == i_drone
            continue;
        end
        
        p_ij = pos(:,i_drone) - pos(:,j);
        dij_ij = norm(p_ij);
        
        if dij_ij > 1e-6
            dd_dp = p_ij;
            
            % Đạo hàm số của beta
            beta_plus = beta_slide(dij_ij + eps_deriv, avoid_params.d_safe, muy);
            beta_minus = beta_slide(dij_ij - eps_deriv, avoid_params.d_safe, muy);
            dbeta_dd = (beta_plus - beta_minus) / (2*eps_deriv);
            
            grad = dPhi_dbeta * dbeta_dd * dd_dp;
            u_avoid = u_avoid - avoid_params.k * grad;
        end
    end
    
    u_h = [0; 0; -prior_params.k_height * (pes(3, i_drone) - pos(3, 1))];


    % =====================================================================
    %  TỔNG HỢP
    % =====================================================================
    u = 5*u_form + u_back + u_damp + 0.5*u_conn + 10*u_avoid + u_h;

end

function beta = beta_slide(dist, d_safe, muy)
    if (dist^2 - d_safe^2) >= 0
        rho = 0;
    else
        rho = 1;
    end
    diff_sq = (dist^2 - d_safe^2)^2;
    beta = (1 - muy * diff_sq / (1 + diff_sq))^rho;
    % Đảm bảo beta không âm
    beta = max(beta, 0);
end

== matlab function Ver1/Drone 10/Pos Estimation ==
  data: p input; v input; pes input; pes_dot output size=[3,1]; params parameter Bus: params_bus
function pes_dot = fcn(p, v, pes, params)

    graph_params = params.graph_params;
    estimation_params = params.estimation_params;

    pes_dot = zeros(3,1);
    
    
    i_drone = 10;  % Drone đang xét
    
    % Reshape input
    pos = reshape(p, graph_params.dim, graph_params.n_drones);
    pes = reshape(pes, graph_params.dim, graph_params.n_drones);
    vel = reshape(v, graph_params.dim, graph_params.n_drones);
    
    % Tính toán gradient term
    grad_term = zeros(graph_params.dim, 1);
    
    n_edges = size(graph_params.edges, 1);
    
    for e = 1:n_edges
        if graph_params.edges(e,1) == i_drone
            j = graph_params.edges(e,2);
        else
            j = graph_params.edges(e,1);
        end

        if j == 1
            grad_term = grad_term + ((pos(:, j) - pes(:,i_drone)) - (pos(:, j) - pos(:, i_drone)));
        else
            grad_term = grad_term + (pes(:, j) - pes(:, i_drone) - (pos(:, j) - pos(:, i_drone)));
        end
    end

    
    % Output
    
    pes_dot1 = vel(:, i_drone) + estimation_params.mu*grad_term;
    pes_dot = [pes_dot1(1); pes_dot1(2); pes_dot1(3)];
end

== matlab function Ver1/Drone 10/Subsystem/Kinematic ==
  data: p_ddot output; u input
function p_ddot = fcn(u)

    p_ddot = u;

end

== matlab function Ver1/Attack Scenario/Attacker ==
  data: pes input; y output; atk_conf input
function y = fcn(pes, atk_conf)

end

== matlab function Ver1/UGV/MATLAB Function ==
  data: u input; psi_dot output
function psi_dot = fcn(u)

    psi_dot = u;
    psi_dot(3) = 0;

end

== matlab function Ver1/UGV/MATLAB Function1 ==
  data: t input; psi_ref output
function psi_ref = fcn(t)

    vx = 20; 

    if t < 20
        psi_ref = zeros(2,1);
    else
        psi_ref = [vx*(t - 20); 10*cos(vx*(t-20))];
    end

end

== matlab function Ver1/Attack Scenario/MATLAB Function ==
  data: p input; d1 output; p0 input; i_min output; n output
function [d1, i_min, n]= fcn(p, p0)
    dmax = 100;
    
    dim = 3;
    n_drones = 10;

    pos = reshape(p, dim, n_drones);

    d1 = norm(pos(:,1) - p0);
    i_min = 1;
    n = 0;
    for i = 1:n_drones
        if norm(pos(:,i) - p0) < d1
            d1 = norm(pos(:,i) - p0);
            i_min = i;
        end
        if norm(pos(:,i) - p0) < dmax
            n = n + 1;
        end
    end
end

== matlab function Ver1/Drone 1/Target Tracking ==
  data: p input; v input; u output; p0 input; n input; gradP output; phi output
function [u, gradP, phi] = observation_barrier_with_desired(p, v, p0, n)
% Hàm thế barrier cho quan sát mục tiêu
% KHÔNG cần vận tốc của mục tiêu (UGV)
% Giữ drone trong khoảng [d_des, d_max]

    % ========== THAM SỐ ==========
    n_drones = 10;
    d_max = 100;            % Tầm quan sát tối đa (m) - KHÔNG ĐƯỢC VƯỢT QUÁ
    d_des = 5;             % Khoảng cách mong muốn (m) - độ cao UAV
    alpha = 2;              % Số mũ
    k_barrier = 5;          % Hệ số khuếch đại
    Kd = 50;                % Damping
    u_max = 20;

    i_drone = 1;
    
    % Điều khiển độ cao (dự phòng)
    altitude_des = d_des;   % Độ cao mong muốn = khoảng cách mong muốn
    K_alt = 3.0;
    
    pos = reshape(p, 3, n_drones);
    vel = reshape(v, 3, n_drones);
    
    % ========== TÁCH THÀNH PHẦN ==========
    r = pos(:, i_drone) - p0;
    d = norm(r);
    
    % Hệ số coverage (khuếch đại khi thiếu quan sát)
    n = max(n, 1);
    coverage = 1 + (1 - n / n_drones);
    
    % ========== LỰC BARRIER THEO PHƯƠNG NGANG ==========
    r_xy = r(1:2);
    d_xy = norm(r_xy);
    
    if d_xy < 1e-6
        F_barrier_xy = zeros(2,1);
        phi_xy = 0;
    else
        % Nếu drone đang ở quá gần (d_xy < d_des) -> cần đẩy ra xa
        if d_xy < d_des
            % Lực đẩy ra xa (để đạt khoảng cách mong muốn)
            phi_xy = k_barrier * coverage * ((d_des - d_xy) / d_des)^2;
            F_barrier_xy = k_barrier * coverage * 2 * (d_des - d_xy) / d_des^2 * (r_xy / d_xy);
        else
            % Barrier function: tiến đến vô cùng khi d_xy → d_max
            if d_xy >= d_max
                % Đã vượt quá tầm quan sát -> lực cực lớn
                phi_xy = k_barrier * coverage * 1e10;
                F_barrier_xy = -1e10 * (r_xy / d_xy);
            else
                xi = (d_xy - d_des) / (d_max - d_des);
                phi_xy = k_barrier * coverage / ((1 - xi)^alpha);
                
                % Đạo hàm dΦ/dξ
                dphi_dxi = k_barrier * coverage * alpha / ((1 - xi)^(alpha+1));
                
                % dξ/dd = 1/(d_max - d_des)
                dphi_dd = dphi_dxi * (1 / (d_max - d_des));
                
                % Lực kéo = -gradient
                F_barrier_xy = -dphi_dd * (r_xy / d_xy);
            end
        end
    end
    
    % ========== DAMPING ==========
    F_damp = -Kd * vel(:, i_drone);
    
    % ========== ĐIỀU KHIỂN ĐỘ CAO (RIÊNG BIỆT) ==========
    p_z = pos(3, i_drone);
    F_alt = -K_alt * (p_z - altitude_des);
    
    % ========== TỔNG HỢP ==========
    u_xy = F_barrier_xy + F_damp(1:2);
    u_z = F_alt + F_damp(3);
    
    u = [u_xy; 0];
    gradP = [F_barrier_xy; 0];
    phi = phi_xy + 0.5 * K_alt * (p_z - altitude_des)^2;
    
end

== matlab function Ver1/Drone 2/Target Tracking ==
  data: p input; v input; u output; p0 input; n input; gradP output; phi output
function [u, gradP, phi] = observation_barrier_with_desired(p, v, p0, n)
% Hàm thế barrier cho quan sát mục tiêu
% KHÔNG cần vận tốc của mục tiêu (UGV)
% Giữ drone trong khoảng [d_des, d_max]

    % ========== THAM SỐ ==========
    n_drones = 10;
    d_max = 100;            % Tầm quan sát tối đa (m) - KHÔNG ĐƯỢC VƯỢT QUÁ
    d_des = 5;             % Khoảng cách mong muốn (m) - độ cao UAV
    alpha = 2;              % Số mũ
    k_barrier = 5;          % Hệ số khuếch đại
    Kd = 50;                % Damping
    u_max = 20;

    i_drone = 2;
    
    % Điều khiển độ cao (dự phòng)
    altitude_des = d_des;   % Độ cao mong muốn = khoảng cách mong muốn
    K_alt = 3.0;
    
    pos = reshape(p, 3, n_drones);
    vel = reshape(v, 3, n_drones);
    
    % ========== TÁCH THÀNH PHẦN ==========
    r = pos(:, i_drone) - p0;
    d = norm(r);
    
    % Hệ số coverage (khuếch đại khi thiếu quan sát)
    n = max(n, 1);
    coverage = 1 + (1 - n / n_drones);
    
    % ========== LỰC BARRIER THEO PHƯƠNG NGANG ==========
    r_xy = r(1:2);
    d_xy = norm(r_xy);
    
    if d_xy < 1e-6
        F_barrier_xy = zeros(2,1);
        phi_xy = 0;
    else
        % Nếu drone đang ở quá gần (d_xy < d_des) -> cần đẩy ra xa
        if d_xy < d_des
            % Lực đẩy ra xa (để đạt khoảng cách mong muốn)
            phi_xy = k_barrier * coverage * ((d_des - d_xy) / d_des)^2;
            F_barrier_xy = k_barrier * coverage * 2 * (d_des - d_xy) / d_des^2 * (r_xy / d_xy);
        else
            % Barrier function: tiến đến vô cùng khi d_xy → d_max
            if d_xy >= d_max
                % Đã vượt quá tầm quan sát -> lực cực lớn
                phi_xy = k_barrier * coverage * 1e10;
                F_barrier_xy = -1e10 * (r_xy / d_xy);
            else
                xi = (d_xy - d_des) / (d_max - d_des);
                phi_xy = k_barrier * coverage / ((1 - xi)^alpha);
                
                % Đạo hàm dΦ/dξ
                dphi_dxi = k_barrier * coverage * alpha / ((1 - xi)^(alpha+1));
                
                % dξ/dd = 1/(d_max - d_des)
                dphi_dd = dphi_dxi * (1 / (d_max - d_des));
                
                % Lực kéo = -gradient
                F_barrier_xy = -dphi_dd * (r_xy / d_xy);
            end
        end
    end
    
    % ========== DAMPING ==========
    F_damp = -Kd * vel(:, i_drone);
    
    % ========== ĐIỀU KHIỂN ĐỘ CAO (RIÊNG BIỆT) ==========
    p_z = pos(3, i_drone);
    F_alt = -K_alt * (p_z - altitude_des);
    
    % ========== TỔNG HỢP ==========
    u_xy = F_barrier_xy + F_damp(1:2);
    u_z = F_alt + F_damp(3);
    
    u = [u_xy; 0];
    gradP = [F_barrier_xy; 0];
    phi = phi_xy + 0.5 * K_alt * (p_z - altitude_des)^2;
    
end
